simulink model "mdaqdemo_can_transmit_HOST"  (R2014a)
settings: Solver=ode3  SolverMode=SingleTasking  StartTime=0.0  StopTime=inf  FixedStep=0.01  RelTol=1e-3
undefined symbols (not defined in the file or in its folder): canChannel
libraries: canlib x2, canmsglib x1
settings Model: CovMetricSettings=dwe  CovHtmlReporting=off  covSaveCumulativeToWorkspaceVar=off  CovSaveSingleToWorkspaceVar=off  CovExternalEMLEnable=on  CovSFcnEnable=on  Creator=skibool  LastModifiedBy=skibool
settings DataIOCC: LimitDataPoints=off  SaveFormat=StructureWithTime
settings DebuggingCC: MergeDetectMultiDrivingBlocksExec=error  SolverPrmCheckMsg=none  FrameProcessingCompatibilityMsg=error  SFUnexpectedBacktrackingDiag=error  SFNoUnconditionalDefaultTransitionDiag=error
settings HardwareCC: ProdBitPerPointer=64  ProdLargestAtomicFloat=Float  ProdIntDivRoundTo=Zero  ProdEndianess=LittleEndian  ProdHWDeviceType=Specified
settings ModelReferenceCC: PropagateSignalLabelsOutOfModel=on
settings GRTTargetCC: TargetLangStandard=C99 (ISO)  GeneratePreprocessorConditionals=Use local settings

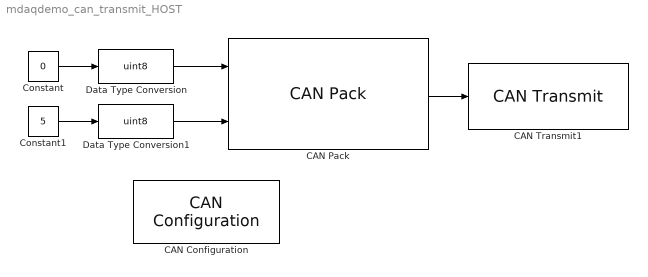
== system mdaqdemo_can_transmit_HOST ==
  CAN Configuration : canlib/CAN Configuration  BlockHandle=46.0023  DeviceMenu=MathWorks Virtual 1 (Channel 1)  Device=Vector VN1640 1 (Channel 2)  ObjConstructor=canChannel('MathWorks','Virtual 1',1)  BusSpeed=500000  EnableBitParameters=off  SJW=1  TSEG1=4  TSEG2=3  NSamples=1  AckMode=Normal
  CAN Pack : canmsglib/CAN Pack  MsgList=(none)  MsgName=CAN Msg  MsgIDType=Standard (11-bit identifier)  MsgIdentifier=1  MsgLength=8  SignalInfo=Signal1$0$8$1$1$1$0$1$0$-Inf$Inf$#Signal2$8$8$1$1$1$0$1$0$-Inf$Inf$#  NSignals=2  StartBits=str2num('[int32(0);int32(8)]')  SignalSizes=str2num('[int32(8);int32(8)]')  ByteOrders=str2num('[int32(1);int32(1)]')  DataTypes=str2num('[int32(1);int32(1)]')  MultiplexTypes=str2num('[int32(1);int32(1)]')  MultiplexValues=str2num('[double(0);double(0)]')  Factors=str2num('[double(1);double(1)]')  Offsets=str2num('[double(0);double(0)]')  Minimums=str2num('[double(-Inf);double(-Inf)]')  Maximums=str2num('[double(Inf);double(Inf)]')  Remote=off  ApplyMinMax=off
      settings: DataFormat=manually specified signals
  CAN Transmit1 : canlib/CAN Transmit  BlockHandle=48.0027  DeviceMenu=MathWorks Virtual 1 (Channel 1)  Device=Vector VN1640 1 (Channel 2)  ObjConstructor=canChannel('MathWorks','Virtual 1',1)  EnablePeriodicTransmit=off  MessagePeriod=1.000
  Constant : Constant  Value=0  SampleTime=-1
  Constant1 : Constant  Value=5  SampleTime=-1
  Data Type Conversion : DataTypeConversion  OutDataTypeStr=uint8
  Data Type Conversion1 : DataTypeConversion  OutDataTypeStr=uint8
  wires:
  CAN Pack/1 -> CAN Transmit1/1
  Constant/1 -> Data Type Conversion/1
  Constant1/1 -> Data Type Conversion1/1
  Data Type Conversion/1 -> CAN Pack/1
  Data Type Conversion1/1 -> CAN Pack/2
